simulink library "NAV420ExLib"  (Simulink 7.3)
settings: Solver=ode45  StartTime=0.0  StopTime=10.0  RelTol=1e-3
libraries: NAV420ExLib_LowLevel x19, NAV420Lib_General_LowLevel x3
settings Model: Creator=djulzz  LastModifiedBy=djulzz

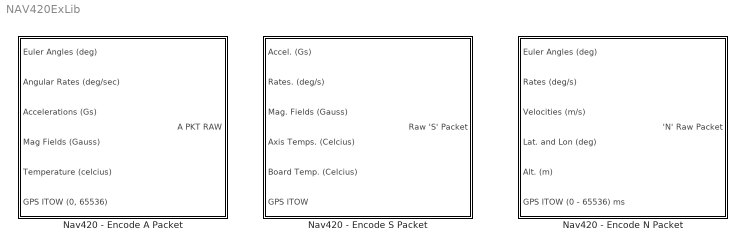
== system NAV420ExLib ==
  Nav420 - Encode A Packet : Subsystem
  Nav420 - Encode N Packet : Subsystem
  Nav420 - Encode S Packet : Subsystem

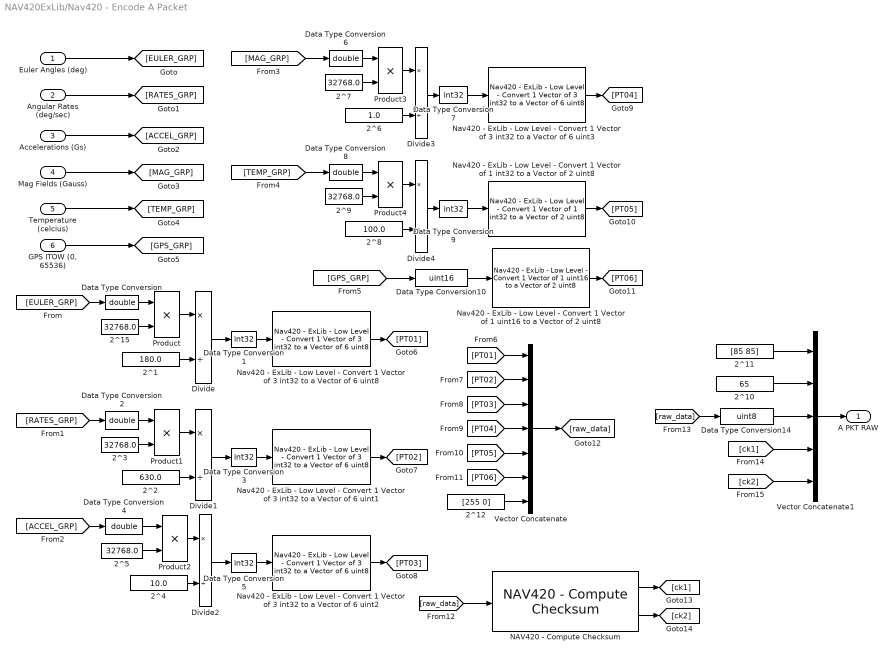
== system NAV420ExLib/Nav420 - Encode A Packet ==
  Euler Angles (deg) : Inport  OutDataType=fixdt(1, 16)  OutScaling=2^0
  Angular Rates (deg/sec) : Inport  Port=2  OutDataType=fixdt(1, 16)  OutScaling=2^0
  Accelerations (Gs) : Inport  Port=3  OutDataType=fixdt(1, 16)  OutScaling=2^0
  Mag Fields (Gauss) : Inport  Port=4  OutDataType=fixdt(1, 16)  OutScaling=2^0
  Temperature (celcius) : Inport  Port=5  OutDataType=fixdt(1, 16)  OutScaling=2^0
  "GPS ITOW (0, 65536)" : Inport  Port=6  DataType=uint16  OutDataType=fixdt(1, 16)  OutScaling=2^0  OutDataTypeStr=uint16
  2^1 : Constant  Value=180.0  OutDataTypeMode=double  OutDataType=fixdt(1, 16)  OutScaling=2^0  OutDataTypeStr=double  SampleTime=-1
  2^10 : Constant  Value=65  OutDataTypeMode=uint8  OutDataType=fixdt(1, 16)  OutScaling=2^0  OutDataTypeStr=uint8  SampleTime=-1
  2^11 : Constant  Value=[85 85]  OutDataTypeMode=uint8  OutDataType=fixdt(1, 16)  OutScaling=2^0  OutDataTypeStr=uint8  SampleTime=-1
  2^12 : Constant  Value=[255 0]  OutDataTypeMode=uint8  OutDataType=fixdt(1, 16)  OutScaling=2^0  OutDataTypeStr=uint8  SampleTime=-1
  2^{3,5,7,9,15} (5 alike) : Constant  Value=32768.0  OutDataTypeMode=double  OutDataType=fixdt(1, 16)  OutScaling=2^0  OutDataTypeStr=double  SampleTime=-1
  2^2 : Constant  Value=630.0  OutDataTypeMode=double  OutDataType=fixdt(1, 16)  OutScaling=2^0  OutDataTypeStr=double  SampleTime=-1
  2^4 : Constant  Value=10.0  OutDataTypeMode=double  OutDataType=fixdt(1, 16)  OutScaling=2^0  OutDataTypeStr=double  SampleTime=-1
  2^6 : Constant  Value=1.0  OutDataTypeMode=double  OutDataType=fixdt(1, 16)  OutScaling=2^0  OutDataTypeStr=double  SampleTime=-1
  2^8 : Constant  Value=100.0  OutDataTypeMode=double  OutDataType=fixdt(1, 16)  OutScaling=2^0  OutDataTypeStr=double  SampleTime=-1
  Data Type Conversion{,2,4,6,8} (5 alike) : DataTypeConversion  OutDataTypeMode=double  OutDataType=fixdt(1, 16)  OutScaling=2^0  OutDataTypeStr=double
  Data Type Conversion{1,3,5,7,9} (5 alike) : DataTypeConversion  OutDataTypeMode=int32  OutDataType=fixdt(1, 16)  OutScaling=2^0  OutDataTypeStr=int32
  Data Type Conversion10 : DataTypeConversion  OutDataTypeMode=uint16  OutDataType=fixdt(1, 16)  OutScaling=2^0  OutDataTypeStr=uint16
  Data Type Conversion14 : DataTypeConversion  OutDataTypeMode=uint8  OutDataType=fixdt(1, 16)  OutScaling=2^0  OutDataTypeStr=uint8
  Divide{,1..4} (5 alike) : Product  Inputs=*/  OutDataType=fixdt(1, 16)  OutScaling=2^-10
  NAV420 - Compute Checksum : NAV420Lib_General_LowLevel/NAV420 - Compute Checksum  SystemSampleTime=-1
  Nav420 - ExLib - Low Level - Convert 1 Vector of 1 int32 to a Vector of 2 uint8 : NAV420ExLib_LowLevel/Nav420 - ExLib - Low Level - Convert 1 Vector of 1 int32 to a Vector of 2 uint8  SystemSampleTime=-1
  Nav420 - ExLib - Low Level - Convert 1 Vector of 1 uint16 to a Vector of 2 uint8 : NAV420ExLib_LowLevel/Nav420 - ExLib - Low Level - Convert 1 Vector of 1 uint16 to a Vector of 2 uint8  SystemSampleTime=-1
  Nav420 - ExLib - Low Level - Convert 1 Vector of 3 int32 to a Vector of 6 uint{1..3,8} (4 alike) : NAV420ExLib_LowLevel/Nav420 - ExLib - Low Level - Convert 1 Vector of 3 int32 to a Vector of 6 uint8  SystemSampleTime=-1
  Product{,1..4} (5 alike) : Product  OutDataType=fixdt(1, 16)  OutScaling=2^0  RndMeth=Zero
  Vector Concatenate : Concatenate  NumInputs=7  Mode=Vector
  Vector Concatenate1 : Concatenate  NumInputs=5  Mode=Vector
  A PKT RAW : Outport  DataType=uint8  OutDataType=fixdt(1, 16)  OutScaling=2^0  OutDataTypeStr=uint8
  wires:
  Euler Angles (deg)/1 -> [EULER_GRP]
  Angular Rates (deg/sec)/1 -> [RATES_GRP]
  Accelerations (Gs)/1 -> [ACCEL_GRP]
  Mag Fields (Gauss)/1 -> [MAG_GRP]
  Temperature (celcius)/1 -> [TEMP_GRP]
  "GPS ITOW (0, 65536)"/1 -> [GPS_GRP]
  [EULER_GRP] -> Data Type Conversion/1
  Data Type Conversion/1 -> Product/1
  2^15/1 -> Product/2
  Product/1 -> Divide/1
  2^1/1 -> Divide/2
  Divide/1 -> Data Type Conversion1/1
  Data Type Conversion2/1 -> Product1/1
  2^3/1 -> Product1/2
  Product1/1 -> Divide1/1
  2^2/1 -> Divide1/2
  Divide1/1 -> Data Type Conversion3/1
  [RATES_GRP] -> Data Type Conversion2/1
  Data Type Conversion4/1 -> Product2/1
  2^5/1 -> Product2/2
  Product2/1 -> Divide2/1
  2^4/1 -> Divide2/2
  Divide2/1 -> Data Type Conversion5/1
  [ACCEL_GRP] -> Data Type Conversion4/1
  Data Type Conversion6/1 -> Product3/1
  2^7/1 -> Product3/2
  Product3/1 -> Divide3/1
  2^6/1 -> Divide3/2
  Divide3/1 -> Data Type Conversion7/1
  [MAG_GRP] -> Data Type Conversion6/1
  2^9/1 -> Product4/2
  Product4/1 -> Divide4/1
  2^8/1 -> Divide4/2
  Divide4/1 -> Data Type Conversion9/1
  Data Type Conversion8/1 -> Product4/1
  [TEMP_GRP] -> Data Type Conversion8/1
  [GPS_GRP] -> Data Type Conversion10/1
  [PT01] -> Vector Concatenate/1
  [PT02] -> Vector Concatenate/2
  [PT03] -> Vector Concatenate/3
  [PT04] -> Vector Concatenate/4
  [PT05] -> Vector Concatenate/5
  [PT06] -> Vector Concatenate/6
  Vector Concatenate/1 -> [raw_data]
  NAV420 - Compute Checksum/2 -> [ck2]
  [raw_data] -> Data Type Conversion14/1
  2^11/1 -> Vector Concatenate1/1
  2^10/1 -> Vector Concatenate1/2
  Data Type Conversion14/1 -> Vector Concatenate1/3
  [ck1] -> Vector Concatenate1/4
  [ck2] -> Vector Concatenate1/5
  Vector Concatenate1/1 -> A PKT RAW/1
  Data Type Conversion1/1 -> Nav420 - ExLib - Low Level - Convert 1 Vector of 3 int32 to a Vector of 6 uint8/1
  Nav420 - ExLib - Low Level - Convert 1 Vector of 3 int32 to a Vector of 6 uint8/1 -> [PT01]
  Data Type Conversion3/1 -> Nav420 - ExLib - Low Level - Convert 1 Vector of 3 int32 to a Vector of 6 uint1/1
  Nav420 - ExLib - Low Level - Convert 1 Vector of 3 int32 to a Vector of 6 uint1/1 -> [PT02]
  Data Type Conversion5/1 -> Nav420 - ExLib - Low Level - Convert 1 Vector of 3 int32 to a Vector of 6 uint2/1
  Nav420 - ExLib - Low Level - Convert 1 Vector of 3 int32 to a Vector of 6 uint2/1 -> [PT03]
  Data Type Conversion7/1 -> Nav420 - ExLib - Low Level - Convert 1 Vector of 3 int32 to a Vector of 6 uint3/1
  Nav420 - ExLib - Low Level - Convert 1 Vector of 3 int32 to a Vector of 6 uint3/1 -> [PT04]
  Data Type Conversion9/1 -> Nav420 - ExLib - Low Level - Convert 1 Vector of 1 int32 to a Vector of 2 uint8/1
  Nav420 - ExLib - Low Level - Convert 1 Vector of 1 int32 to a Vector of 2 uint8/1 -> [PT05]
  Data Type Conversion10/1 -> Nav420 - ExLib - Low Level - Convert 1 Vector of 1 uint16 to a Vector of 2 uint8/1
  Nav420 - ExLib - Low Level - Convert 1 Vector of 1 uint16 to a Vector of 2 uint8/1 -> [PT06]
  2^12/1 -> Vector Concatenate/7
  [raw_data] -> NAV420 - Compute Checksum/1
  NAV420 - Compute Checksum/1 -> [ck1]

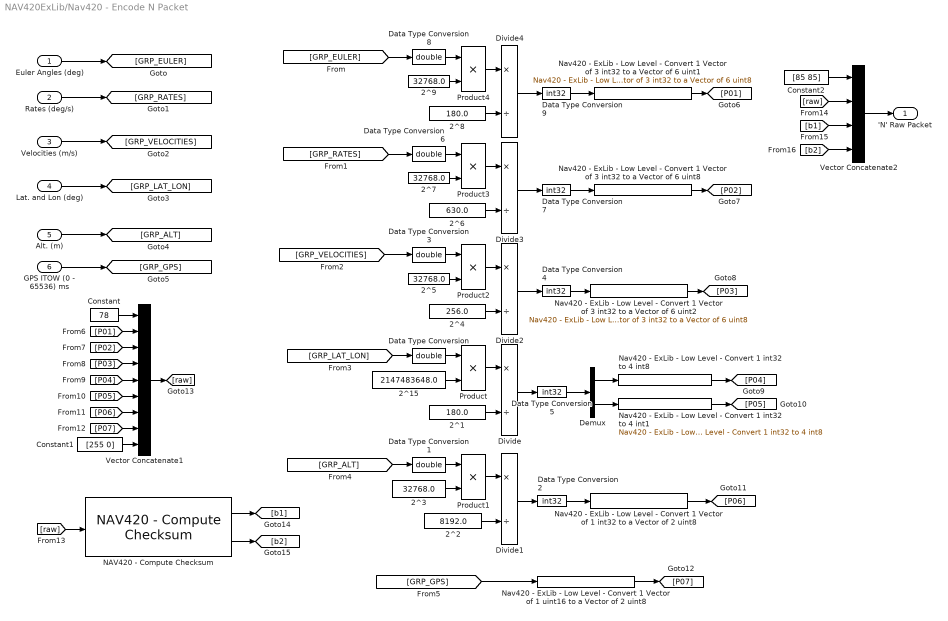
== system NAV420ExLib/Nav420 - Encode N Packet ==
  Euler Angles (deg) : Inport  DataType=double  OutDataType=fixdt(1, 16)  OutScaling=2^0  OutDataTypeStr=double
  Rates (deg/s) : Inport  Port=2  DataType=double  OutDataType=fixdt(1, 16)  OutScaling=2^0  OutDataTypeStr=double
  Velocities (m/s) : Inport  Port=3  DataType=double  OutDataType=fixdt(1, 16)  OutScaling=2^0  OutDataTypeStr=double
  Lat. and Lon (deg) : Inport  Port=4  DataType=double  OutDataType=fixdt(1, 16)  OutScaling=2^0  OutDataTypeStr=double
  Alt. (m) : Inport  Port=5  DataType=double  OutDataType=fixdt(1, 16)  OutScaling=2^0  OutDataTypeStr=double
  GPS ITOW (0 - 65536) ms : Inport  Port=6  DataType=uint16  OutDataType=fixdt(1, 16)  OutScaling=2^0  OutDataTypeStr=uint16
  2^1 : Constant  Value=180.0  OutDataTypeMode=double  OutDataType=fixdt(1, 16)  OutScaling=2^0  OutDataTypeStr=double  SampleTime=-1
  2^15 : Constant  Value=2147483648.0  OutDataTypeMode=double  OutDataType=fixdt(1, 16)  OutScaling=2^0  OutDataTypeStr=double  SampleTime=-1
  2^2 : Constant  Value=8192.0  OutDataTypeMode=double  OutDataType=fixdt(1, 16)  OutScaling=2^0  OutDataTypeStr=double  SampleTime=-1
  2^{3,5,7,9} (4 alike) : Constant  Value=32768.0  OutDataTypeMode=double  OutDataType=fixdt(1, 16)  OutScaling=2^0  OutDataTypeStr=double  SampleTime=-1
  2^4 : Constant  Value=256.0  OutDataTypeMode=double  OutDataType=fixdt(1, 16)  OutScaling=2^0  OutDataTypeStr=double  SampleTime=-1
  2^6 : Constant  Value=630.0  OutDataTypeMode=double  OutDataType=fixdt(1, 16)  OutScaling=2^0  OutDataTypeStr=double  SampleTime=-1
  2^8 : Constant  Value=180.0  OutDataTypeMode=double  OutDataType=fixdt(1, 16)  OutScaling=2^0  OutDataTypeStr=double  SampleTime=-1
  Constant : Constant  Value=78  OutDataTypeMode=uint8  OutDataType=fixdt(1, 16)  OutScaling=2^0  OutDataTypeStr=uint8  SampleTime=-1
  Constant1 : Constant  Value=[255 0]  OutDataTypeMode=uint8  OutDataType=fixdt(1, 16)  OutScaling=2^0  OutDataTypeStr=uint8  SampleTime=-1
  Constant2 : Constant  Value=[85 85]  OutDataTypeMode=uint8  OutDataType=fixdt(1, 16)  OutScaling=2^0  OutDataTypeStr=uint8  SampleTime=-1
  Data Type Conversion{,1,3,6,8} (5 alike) : DataTypeConversion  OutDataTypeMode=double  OutDataType=fixdt(1, 16)  OutScaling=2^0  OutDataTypeStr=double
  Data Type Conversion{2,4..5,7,9} (5 alike) : DataTypeConversion  OutDataTypeMode=int32  OutDataType=fixdt(1, 16)  OutScaling=2^0  OutDataTypeStr=int32
  Demux : Demux  Outputs=2
  Divide{,1..4} (5 alike) : Product  Inputs=*/  OutDataType=fixdt(1, 16)  OutScaling=2^-10
  NAV420 - Compute Checksum : NAV420Lib_General_LowLevel/NAV420 - Compute Checksum  SystemSampleTime=-1
  Nav420 - ExLib - Low Level - Convert 1 Vector of 1 int32 to a Vector of 2 uint8 : NAV420ExLib_LowLevel/Nav420 - ExLib - Low Level - Convert 1 Vector of 1 int32 to a Vector of 2 uint8  SystemSampleTime=-1
  Nav420 - ExLib - Low Level - Convert 1 Vector of 1 uint16 to a Vector of 2 uint8 : NAV420ExLib_LowLevel/Nav420 - ExLib - Low Level - Convert 1 Vector of 1 uint16 to a Vector of 2 uint8  SystemSampleTime=-1
  Nav420 - ExLib - Low Level - Convert 1 Vector of 3 int32 to a Vector of 6 uint1 : NAV420ExLib_LowLevel/Nav420 - ExLib - Low Level - Convert 1 Vector of 3 int32 to a Vector of 6 uint8  SystemSampleTime=-1
  Nav420 - ExLib - Low Level - Convert 1 Vector of 3 int32 to a Vector of 6 uint2 : NAV420ExLib_LowLevel/Nav420 - ExLib - Low Level - Convert 1 Vector of 3 int32 to a Vector of 6 uint8  SystemSampleTime=-1
  Nav420 - ExLib - Low Level - Convert 1 Vector of 3 int32 to a Vector of 6 uint8 : NAV420ExLib_LowLevel/Nav420 - ExLib - Low Level - Convert 1 Vector of 3 int32 to a Vector of 6 uint8  SystemSampleTime=-1
  Nav420 - ExLib - Low Level - Convert 1 int32 to 4 int1 : NAV420ExLib_LowLevel/Nav420 - ExLib - Low Level - Convert 1 int32 to 4 int8  SystemSampleTime=-1
  Nav420 - ExLib - Low Level - Convert 1 int32 to 4 int8 : NAV420ExLib_LowLevel/Nav420 - ExLib - Low Level - Convert 1 int32 to 4 int8  SystemSampleTime=-1
  Product{,1..4} (5 alike) : Product  OutDataType=fixdt(1, 16)  OutScaling=2^0  RndMeth=Zero
  Vector Concatenate1 : Concatenate  NumInputs=9  Mode=Vector
  Vector Concatenate2 : Concatenate  NumInputs=4  Mode=Vector
  'N' Raw Packet : Outport  DataType=uint8  OutDataType=fixdt(1, 16)  OutScaling=2^0  OutDataTypeStr=uint8
  wires:
  Euler Angles (deg)/1 -> [GRP_EULER]
  Rates (deg/s)/1 -> [GRP_RATES]
  Velocities (m/s)/1 -> [GRP_VELOCITIES]
  Lat. and Lon (deg)/1 -> [GRP_LAT_LON]
  Alt. (m)/1 -> [GRP_ALT]
  GPS ITOW (0 - 65536) ms/1 -> [GRP_GPS]
  Demux/1 -> Nav420 - ExLib - Low Level - Convert 1 int32 to 4 int8/1
  Demux/2 -> Nav420 - ExLib - Low Level - Convert 1 int32 to 4 int1/1
  Data Type Conversion/1 -> Product/1
  2^15/1 -> Product/2
  Product/1 -> Divide/1
  2^1/1 -> Divide/2
  Divide/1 -> Data Type Conversion5/1
  [GRP_LAT_LON] -> Data Type Conversion/1
  Data Type Conversion5/1 -> Demux/1
  Data Type Conversion1/1 -> Product1/1
  2^3/1 -> Product1/2
  Product1/1 -> Divide1/1
  2^2/1 -> Divide1/2
  Divide1/1 -> Data Type Conversion2/1
  Data Type Conversion2/1 -> Nav420 - ExLib - Low Level - Convert 1 Vector of 1 int32 to a Vector of 2 uint8/1
  [GRP_ALT] -> Data Type Conversion1/1
  [GRP_GPS] -> Nav420 - ExLib - Low Level - Convert 1 Vector of 1 uint16 to a Vector of 2 uint8/1
  Data Type Conversion3/1 -> Product2/1
  2^5/1 -> Product2/2
  Product2/1 -> Divide2/1
  2^4/1 -> Divide2/2
  [GRP_VELOCITIES] -> Data Type Conversion3/1
  Divide2/1 -> Data Type Conversion4/1
  Data Type Conversion4/1 -> Nav420 - ExLib - Low Level - Convert 1 Vector of 3 int32 to a Vector of 6 uint2/1
  Data Type Conversion6/1 -> Product3/1
  2^7/1 -> Product3/2
  Product3/1 -> Divide3/1
  2^6/1 -> Divide3/2
  Divide3/1 -> Data Type Conversion7/1
  [GRP_RATES] -> Data Type Conversion6/1
  Data Type Conversion7/1 -> Nav420 - ExLib - Low Level - Convert 1 Vector of 3 int32 to a Vector of 6 uint8/1
  Data Type Conversion8/1 -> Product4/1
  2^9/1 -> Product4/2
  Product4/1 -> Divide4/1
  2^8/1 -> Divide4/2
  Divide4/1 -> Data Type Conversion9/1
  Data Type Conversion9/1 -> Nav420 - ExLib - Low Level - Convert 1 Vector of 3 int32 to a Vector of 6 uint1/1
  [GRP_EULER] -> Data Type Conversion8/1
  Nav420 - ExLib - Low Level - Convert 1 Vector of 3 int32 to a Vector of 6 uint1/1 -> [P01]
  Nav420 - ExLib - Low Level - Convert 1 Vector of 3 int32 to a Vector of 6 uint8/1 -> [P02]
  Nav420 - ExLib - Low Level - Convert 1 Vector of 3 int32 to a Vector of 6 uint2/1 -> [P03]
  Nav420 - ExLib - Low Level - Convert 1 int32 to 4 int8/1 -> [P04]
  Nav420 - ExLib - Low Level - Convert 1 int32 to 4 int1/1 -> [P05]
  Nav420 - ExLib - Low Level - Convert 1 Vector of 1 int32 to a Vector of 2 uint8/1 -> [P06]
  Nav420 - ExLib - Low Level - Convert 1 Vector of 1 uint16 to a Vector of 2 uint8/1 -> [P07]
  Constant/1 -> Vector Concatenate1/1
  [P01] -> Vector Concatenate1/2
  Constant1/1 -> Vector Concatenate1/9
  [P07] -> Vector Concatenate1/8
  [P06] -> Vector Concatenate1/7
  [P05] -> Vector Concatenate1/6
  [P04] -> Vector Concatenate1/5
  [P03] -> Vector Concatenate1/4
  [P02] -> Vector Concatenate1/3
  Vector Concatenate1/1 -> [raw]
  [raw] -> NAV420 - Compute Checksum/1
  NAV420 - Compute Checksum/2 -> [b2]
  NAV420 - Compute Checksum/1 -> [b1]
  Constant2/1 -> Vector Concatenate2/1
  [raw] -> Vector Concatenate2/2
  [b1] -> Vector Concatenate2/3
  [b2] -> Vector Concatenate2/4
  Vector Concatenate2/1 -> 'N' Raw Packet/1

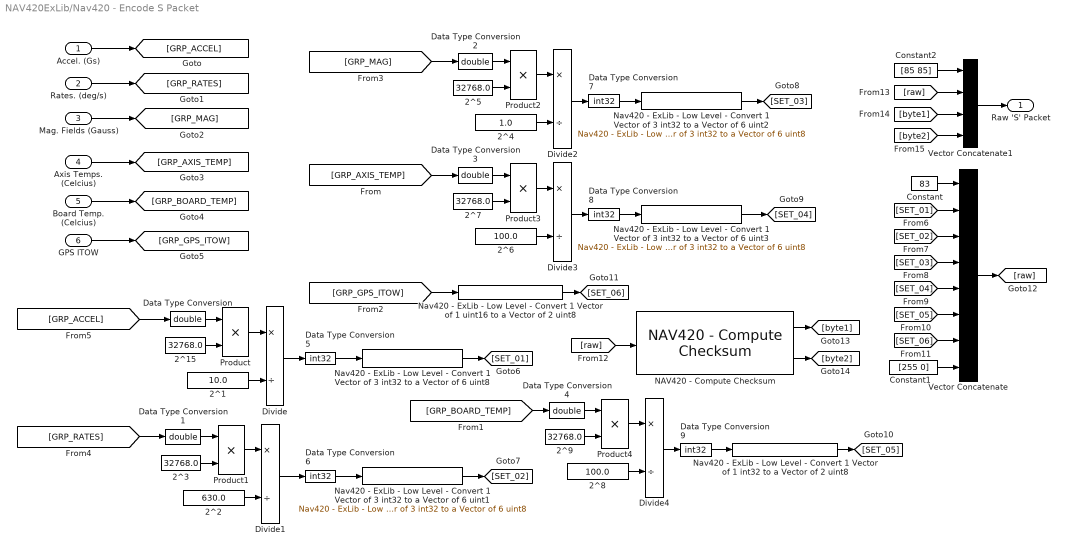
== system NAV420ExLib/Nav420 - Encode S Packet ==
  Accel. (Gs) : Inport  DataType=double  OutDataType=fixdt(1, 16)  OutScaling=2^0  OutDataTypeStr=double
  Rates. (deg/s) : Inport  Port=2  DataType=double  OutDataType=fixdt(1, 16)  OutScaling=2^0  OutDataTypeStr=double
  Mag. Fields (Gauss) : Inport  Port=3  DataType=double  OutDataType=fixdt(1, 16)  OutScaling=2^0  OutDataTypeStr=double
  Axis Temps. (Celcius) : Inport  Port=4  DataType=double  OutDataType=fixdt(1, 16)  OutScaling=2^0  OutDataTypeStr=double
  Board Temp. (Celcius) : Inport  Port=5  DataType=double  OutDataType=fixdt(1, 16)  OutScaling=2^0  OutDataTypeStr=double
  GPS ITOW : Inport  Port=6  DataType=uint16  OutDataType=fixdt(1, 16)  OutScaling=2^0  OutDataTypeStr=uint16
  2^1 : Constant  Value=10.0  OutDataTypeMode=double  OutDataType=fixdt(1, 16)  OutScaling=2^0  OutDataTypeStr=double  SampleTime=-1
  2^{3,5,7,9,15} (5 alike) : Constant  Value=32768.0  OutDataTypeMode=double  OutDataType=fixdt(1, 16)  OutScaling=2^0  OutDataTypeStr=double  SampleTime=-1
  2^2 : Constant  Value=630.0  OutDataTypeMode=double  OutDataType=fixdt(1, 16)  OutScaling=2^0  OutDataTypeStr=double  SampleTime=-1
  2^4 : Constant  Value=1.0  OutDataTypeMode=double  OutDataType=fixdt(1, 16)  OutScaling=2^0  OutDataTypeStr=double  SampleTime=-1
  2^6 : Constant  Value=100.0  OutDataTypeMode=double  OutDataType=fixdt(1, 16)  OutScaling=2^0  OutDataTypeStr=double  SampleTime=-1
  2^8 : Constant  Value=100.0  OutDataTypeMode=double  OutDataType=fixdt(1, 16)  OutScaling=2^0  OutDataTypeStr=double  SampleTime=-1
  Constant : Constant  Value=83  OutDataTypeMode=uint8  OutDataType=fixdt(1, 16)  OutScaling=2^0  OutDataTypeStr=uint8  SampleTime=-1
  Constant1 : Constant  Value=[255 0]  OutDataTypeMode=uint8  OutDataType=fixdt(1, 16)  OutScaling=2^0  OutDataTypeStr=uint8  SampleTime=-1
  Constant2 : Constant  Value=[85 85]  OutDataTypeMode=uint8  OutDataType=fixdt(1, 16)  OutScaling=2^0  OutDataTypeStr=uint8  SampleTime=-1
  Data Type Conversion{,1..4} (5 alike) : DataTypeConversion  OutDataTypeMode=double  OutDataType=fixdt(1, 16)  OutScaling=2^0  OutDataTypeStr=double
  Data Type Conversion{5..9} (5 alike) : DataTypeConversion  OutDataTypeMode=int32  OutDataType=fixdt(1, 16)  OutScaling=2^0  OutDataTypeStr=int32
  Divide{,1..4} (5 alike) : Product  Inputs=*/  OutDataType=fixdt(1, 16)  OutScaling=2^-10
  NAV420 - Compute Checksum : NAV420Lib_General_LowLevel/NAV420 - Compute Checksum  SystemSampleTime=-1
  Nav420 - ExLib - Low Level - Convert 1 Vector of 1 int32 to a Vector of 2 uint8 : NAV420ExLib_LowLevel/Nav420 - ExLib - Low Level - Convert 1 Vector of 1 int32 to a Vector of 2 uint8  SystemSampleTime=-1
  Nav420 - ExLib - Low Level - Convert 1 Vector of 1 uint16 to a Vector of 2 uint8 : NAV420ExLib_LowLevel/Nav420 - ExLib - Low Level - Convert 1 Vector of 1 uint16 to a Vector of 2 uint8  SystemSampleTime=-1
  Nav420 - ExLib - Low Level - Convert 1 Vector of 3 int32 to a Vector of 6 uint{1..3,8} (4 alike) : NAV420ExLib_LowLevel/Nav420 - ExLib - Low Level - Convert 1 Vector of 3 int32 to a Vector of 6 uint8  SystemSampleTime=-1
  Product{,1..4} (5 alike) : Product  OutDataType=fixdt(1, 16)  OutScaling=2^0  RndMeth=Zero
  Vector Concatenate : Concatenate  NumInputs=8  Mode=Vector
  Vector Concatenate1 : Concatenate  NumInputs=4  Mode=Vector
  Raw 'S' Packet : Outport  OutDataType=fixdt(1, 16)  OutScaling=2^0
  wires:
  Accel. (Gs)/1 -> [GRP_ACCEL]
  Rates. (deg/s)/1 -> [GRP_RATES]
  Mag. Fields (Gauss)/1 -> [GRP_MAG]
  Axis Temps. (Celcius)/1 -> [GRP_AXIS_TEMP]
  Board Temp. (Celcius)/1 -> [GRP_BOARD_TEMP]
  GPS ITOW/1 -> [GRP_GPS_ITOW]
  Data Type Conversion/1 -> Product/1
  2^15/1 -> Product/2
  Product/1 -> Divide/1
  2^1/1 -> Divide/2
  [GRP_ACCEL] -> Data Type Conversion/1
  Data Type Conversion1/1 -> Product1/1
  2^3/1 -> Product1/2
  Product1/1 -> Divide1/1
  2^2/1 -> Divide1/2
  [GRP_RATES] -> Data Type Conversion1/1
  Data Type Conversion2/1 -> Product2/1
  2^5/1 -> Product2/2
  Product2/1 -> Divide2/1
  2^4/1 -> Divide2/2
  [GRP_MAG] -> Data Type Conversion2/1
  Data Type Conversion3/1 -> Product3/1
  2^7/1 -> Product3/2
  Product3/1 -> Divide3/1
  2^6/1 -> Divide3/2
  [GRP_AXIS_TEMP] -> Data Type Conversion3/1
  Data Type Conversion4/1 -> Product4/1
  2^9/1 -> Product4/2
  Product4/1 -> Divide4/1
  2^8/1 -> Divide4/2
  [GRP_BOARD_TEMP] -> Data Type Conversion4/1
  Divide/1 -> Data Type Conversion5/1
  Divide1/1 -> Data Type Conversion6/1
  Divide2/1 -> Data Type Conversion7/1
  Divide3/1 -> Data Type Conversion8/1
  Divide4/1 -> Data Type Conversion9/1
  Data Type Conversion5/1 -> Nav420 - ExLib - Low Level - Convert 1 Vector of 3 int32 to a Vector of 6 uint8/1
  Data Type Conversion6/1 -> Nav420 - ExLib - Low Level - Convert 1 Vector of 3 int32 to a Vector of 6 uint1/1
  Data Type Conversion7/1 -> Nav420 - ExLib - Low Level - Convert 1 Vector of 3 int32 to a Vector of 6 uint2/1
  Data Type Conversion8/1 -> Nav420 - ExLib - Low Level - Convert 1 Vector of 3 int32 to a Vector of 6 uint3/1
  Data Type Conversion9/1 -> Nav420 - ExLib - Low Level - Convert 1 Vector of 1 int32 to a Vector of 2 uint8/1
  [GRP_GPS_ITOW] -> Nav420 - ExLib - Low Level - Convert 1 Vector of 1 uint16 to a Vector of 2 uint8/1
  Nav420 - ExLib - Low Level - Convert 1 Vector of 3 int32 to a Vector of 6 uint8/1 -> [SET_01]
  Nav420 - ExLib - Low Level - Convert 1 Vector of 3 int32 to a Vector of 6 uint1/1 -> [SET_02]
  Nav420 - ExLib - Low Level - Convert 1 Vector of 3 int32 to a Vector of 6 uint2/1 -> [SET_03]
  Nav420 - ExLib - Low Level - Convert 1 Vector of 3 int32 to a Vector of 6 uint3/1 -> [SET_04]
  Nav420 - ExLib - Low Level - Convert 1 Vector of 1 int32 to a Vector of 2 uint8/1 -> [SET_05]
  Nav420 - ExLib - Low Level - Convert 1 Vector of 1 uint16 to a Vector of 2 uint8/1 -> [SET_06]
  Constant/1 -> Vector Concatenate/1
  [SET_01] -> Vector Concatenate/2
  [SET_02] -> Vector Concatenate/3
  [SET_03] -> Vector Concatenate/4
  [SET_04] -> Vector Concatenate/5
  [SET_05] -> Vector Concatenate/6
  [SET_06] -> Vector Concatenate/7
  Constant1/1 -> Vector Concatenate/8
  Vector Concatenate/1 -> [raw]
  [raw] -> NAV420 - Compute Checksum/1
  NAV420 - Compute Checksum/1 -> [byte1]
  NAV420 - Compute Checksum/2 -> [byte2]
  Constant2/1 -> Vector Concatenate1/1
  [raw] -> Vector Concatenate1/2
  [byte1] -> Vector Concatenate1/3
  [byte2] -> Vector Concatenate1/4
  Vector Concatenate1/1 -> Raw 'S' Packet/1
